simulink library "solar_panel_power_lib"  (R2016b)
settings: Solver=VariableStepAuto  StartTime=0.0  StopTime=10.0  RelTol=1e-3
undefined symbols (not defined in the file): sim_params
libraries: aerolibutil x1
settings Model: Creator=taylorreynolds  LastModifiedBy=Taylor

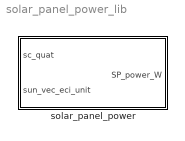
== system solar_panel_power_lib ==
  solar_panel_power : Subsystem

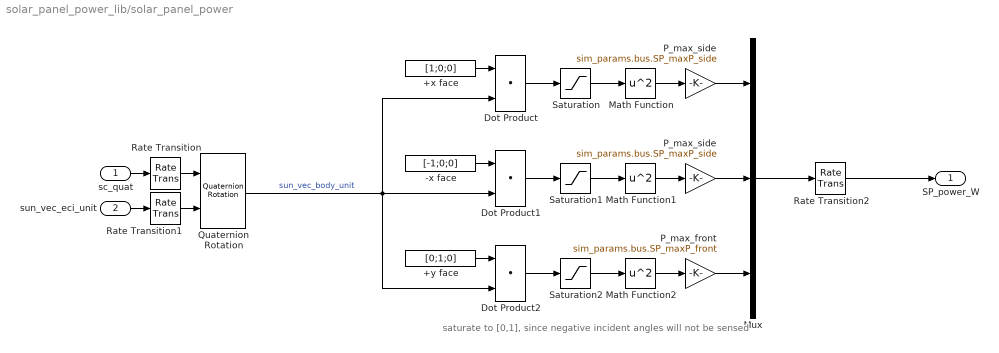
== system solar_panel_power_lib/solar_panel_power ==
  note: saturate to [0,1], since negative incident angles will not be sensed
  sc_quat : Inport
  sun_vec_eci_unit : Inport  Port=2
  +x face : Constant  Value=[1;0;0]  SampleTime=sim_params.sample_time_s
  +y face : Constant  Value=[0;1;0]  SampleTime=sim_params.sample_time_s
  -x face : Constant  Value=[-1;0;0]  SampleTime=sim_params.sample_time_s
  Dot Product : DotProduct  InputSameDT=on  OutDataTypeStr=Inherit: Inherit via internal rule
  Dot Product1 : DotProduct  InputSameDT=on  OutDataTypeStr=Inherit: Inherit via internal rule
  Dot Product2 : DotProduct  InputSameDT=on  OutDataTypeStr=Inherit: Inherit via internal rule
  Math Function : Math  Operator=square  SaturateOnIntegerOverflow=on
  Math Function1 : Math  Operator=square  SaturateOnIntegerOverflow=on
  Math Function2 : Math  Operator=square  SaturateOnIntegerOverflow=on
  Mux : Mux  Inputs=3
  P_max_front : Gain  Gain=sim_params.bus.SP_maxP_front
  P_max_side : Gain  Gain=sim_params.bus.SP_maxP_side
  "P_max_side " : Gain  Gain=sim_params.bus.SP_maxP_side
  Quaternion Rotation : aerolibutil/Quaternion Rotation
  Rate Transition : RateTransition  X0=[1;0;0;0]  OutPortSampleTime=sim_params.sample_time_s
  Rate Transition1 : RateTransition  OutPortSampleTime=sim_params.sample_time_s
  Rate Transition2 : RateTransition
  Saturation : Saturate  UpperLimit=1  LowerLimit=0
  Saturation1 : Saturate  UpperLimit=1  LowerLimit=0
  Saturation2 : Saturate  UpperLimit=1  LowerLimit=0
  SP_power_W : Outport
  wires:
  sun_vec_eci_unit/1 -> Rate Transition1/1
  sc_quat/1 -> Rate Transition/1
  Quaternion Rotation/1 -> Dot Product/2, Dot Product1/2, Dot Product2/2  "sun_vec_body_unit"
  +x face/1 -> Dot Product/1
  -x face/1 -> Dot Product1/1
  +y face/1 -> Dot Product2/1
  Dot Product/1 -> Saturation/1
  Dot Product1/1 -> Saturation1/1
  Dot Product2/1 -> Saturation2/1
  Saturation/1 -> Math Function/1
  Saturation1/1 -> Math Function1/1
  Saturation2/1 -> Math Function2/1
  Math Function/1 -> P_max_side/1
  Math Function1/1 -> "P_max_side "/1
  Math Function2/1 -> P_max_front/1
  P_max_side/1 -> Mux/1
  "P_max_side "/1 -> Mux/2
  P_max_front/1 -> Mux/3
  Mux/1 -> Rate Transition2/1
  Rate Transition/1 -> Quaternion Rotation/1
  Rate Transition1/1 -> Quaternion Rotation/2
  Rate Transition2/1 -> SP_power_W/1
